simulink model "NHS_simulink_1024nfft_buffer_2017a"  (R2017a)
settings: Solver=FixedStepDiscrete  StartTime=0.0  StopTime=inf  RelTol=1e-3
libraries: simulink x2, audiosources x1, dspsnks4 x1, dspxfrm3 x1, dspvision x1
settings Model: Creator=zhouyiliang  LastModifiedBy=zhouyiliang
settings SolverCC: AutoInsertRateTranBlk=on
settings DataIOCC: LimitDataPoints=on  SaveOutput=off  SignalLogging=off  SaveTime=off  ReturnWorkspaceOutputs=on
settings OptimizationCC: LifeSpan=inf
settings DebuggingCC: AlgebraicLoopMsg=error  SingleTaskRateTransMsg=error  AllowSymbolicDim=off  SFUnexpectedBacktrackingDiag=warning  SFNoUnconditionalDefaultTransitionDiag=warning  SFExecutionAtInitializationDiag=none
settings GRTTargetCC: TargetLangStandard=C89/C90 (ANSI)
settings ConfigComp: CovMetricSettings=dw  CovSaveCumulativeToWorkspaceVar=on  CovSaveSingleToWorkspaceVar=on  CovExternalEMLEnable=off  CovSFcnEnable=off

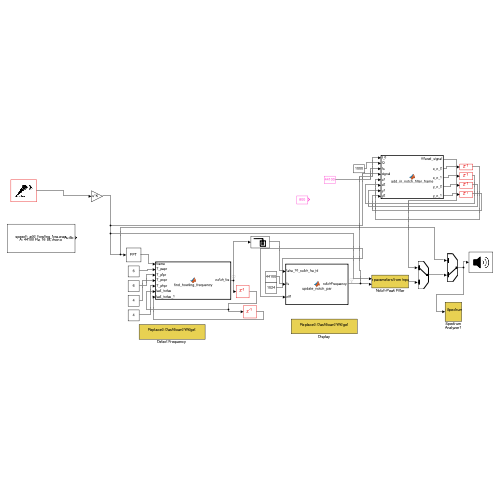
[thumbnail: Simulink's stored preview of the top-level diagram]
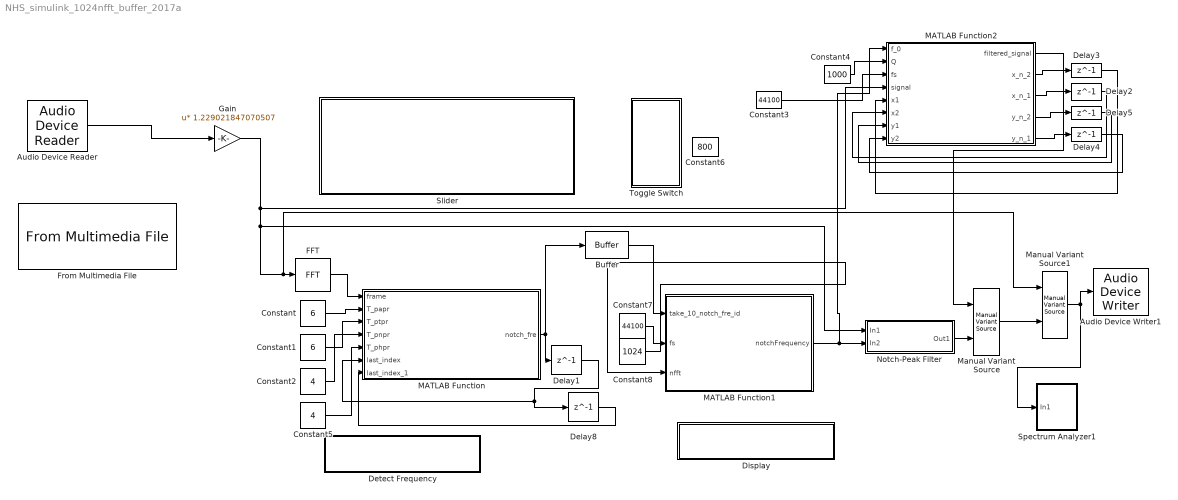
== system NHS_simulink_1024nfft_buffer_2017a ==
  Audio Device Reader : audiosources/Audio Device Reader  Driver=CoreAudio  Device=External Microphone  SampleRate=44100  NumChannels=1  SamplesPerFrame=882  BitDepth=16-bit integer  NumBuffers=10  DefaultInputChannelMapping=on  InputChannelMapping=1:2  OutputNumOverrunSamples=off  OutputDataType=double  DriverIdx=5  DeviceWarnFlag=''
  Audio Device Writer1 : dspsnks4/Audio Device Writer  Driver=CoreAudio  Device=External Headphones  InheritSampleRate=on  SampleRate=44100  BitDepth=16-bit integer  BufferSize=4096  NumBuffers=10  DefaultOutputChannelMapping=on  OutputChannelMapping=1:2  OutputNumUnderrunSamples=off  DriverIdx=5  DeviceWarnFlag=''
  Buffer : Buffer  N=5  OutputFrames=off
  Constant : Constant  Value=6
  Constant1 : Constant  Value=6
  Constant2 : Constant  Value=4
  Constant3 : Constant  Value=44100
  Constant4 : Constant  Value=1000
  Constant5 : Constant  Value=4
  Constant6 : Constant  Value=800
  Constant7 : Constant  Value=44100
  Constant8 : Constant  Value=1024
  Delay{1..5,8} (6 alike) : Delay  DelayLength=1  InitialCondition=0
  "Detect Frequency " : Subsystem  Description=Replaced Block  mask(Replaced Block){}
      mask help: This block has been replaced with an empty subsystem because it used functionality that is unavailable in Simulink R2017a.
      mask Display: fprintf('Replaced: %s\n','Dashboard Widget')
  Display : Subsystem  Description=Replaced Block  mask(Replaced Block){}
      mask help: This block has been replaced with an empty subsystem because it used functionality that is unavailable in Simulink R2017a.
      mask Display: fprintf('Replaced: %s\n','Dashboard Widget')
  FFT : dspxfrm3/FFT  FFTImplementation=Auto  CompMethod=Table lookup  TableOpt=NEW  TableOptActive=Speed  BitRevOrder=off  Normalize=off  InheritFFTLength=off  FFTLength=1024  WrapInput=on  roundingMode=Floor  overflowMode=off  firstCoeffDataTypeStr=Inherit: Same word length as input  firstCoeffLastDataTypeStr=Inherit: Same word length as input  outputMin=[]  outputMax=[]
  From Multimedia File : dspvision/From Multimedia File  inputFilename=/Users/zhouyiliang/Desktop/work/sound_output/speech_add_howling_fyra.wav  loop=on  numPlays=inf  outputStreams=Audio only  videoDataType=single  audioDataType=double  inheritSampleTime=on  userDefinedSampleTime=1/30  noAudioOutput=off  isIntensityVideo=off  fourcc=RGB  colorVideoFormat=Separate color signals  outputEOF=off  dataOrg=Column-major  audioFrameSize=882  computeAudioFrameSize=off  outSamplingMode=Sample based
  Gain : Gain  Gain=1.229021847070507  Multiplication=Matrix(u*K)
  MATLAB Function : MATLAB Function  TreatAsAtomicUnit=on
  MATLAB Function1 : MATLAB Function  TreatAsAtomicUnit=on
  MATLAB Function2 : MATLAB Function  TreatAsAtomicUnit=on
  Manual Variant Source : simulink/Signal Routing/Manual Variant Source  NumChoices=2  OverrideUsingVariant=V_1
  Manual Variant Source1 : simulink/Signal Routing/Manual Variant Source  NumChoices=2  OverrideUsingVariant=V_2
  Notch-Peak Filter : Subsystem  Description=Replaced Block  InitFcn=error('This block was designed with a newer version of Simulink. Unfortunately, your Simulink version does not support these features.')  mask(Replaced Block){}
      mask help: This block has been replaced with an empty subsystem because it used functionality that is unavailable in Simulink R2017a.
      mask Display: fprintf('Replaced: %s\n','Specifying tunable parameters from input ports supported in R2018a')
  Slider : Subsystem  DialogController=hmiCreateDDGDialog  IsWebBlock=on  mask(MWDashboardBlock){webBlockId=bec0057f-2732-4f60-8ecc-0ddb8d2f5a2f, webBlockType=slider, ShowInLibBrowser=on, ShowInitialText=on, HMISrcModelName=NHS_simulink_1024nfft_buffer_2017a}
      mask prompts: webBlockId "WebBlock Id"; webBlockType "WebBlock Type"; HMISrcModelName "Source Model"
      mask help: Set value to tune parameters or variables.
      mask Help: helpview([docroot '/mapfiles/simulink.map'], 'hmi_slider')
      mask Display:
      | if strcmp(get_param(bdroot(gcb),'BlockDiagramType'),'library')
      |  image([(matlabroot) '/toolbox/simulink/hmi/icons/Slider.png'])
      | end
  Spectrum Analyzer1 : Subsystem  Description=Replaced Block  mask(Replaced Block){}
      mask help: This block has been replaced with an empty subsystem because it used functionality that is unavailable in Simulink R2017a.
      mask Display: fprintf('Replaced: %s\n','SpectrumAnalyzer')
  Toggle Switch : Subsystem  DialogController=hmiCreateDDGDialog  IsWebBlock=on  mask(MWDashboardBlock){webBlockId=04cc992a-a373-4357-83c5-108d627a7a1e, webBlockType=toggleswitch, ShowInLibBrowser=on, ShowInitialText=on, HMISrcModelName=NHS_simulink_1024nfft_buffer_2017a}
      mask prompts: webBlockId "WebBlock Id"; webBlockType "WebBlock Type"; HMISrcModelName "Source Model"
      mask help: Set on/off value to tune parameters or variables.
      mask Help: helpview([docroot '/mapfiles/simulink.map'], 'hmi_switch')
      mask Display:
      | if strcmp(get_param(bdroot(gcb),'BlockDiagramType'),'library')
      |  image([(matlabroot) '/toolbox/simulink/hmi/icons/ToggleSwitch.png'])
      | end
  wires:
  FFT/1 -> MATLAB Function/1(frame)
  Constant/1 -> MATLAB Function/2(T_papr)
  Constant1/1 -> MATLAB Function/3(T_ptpr)
  Constant2/1 -> MATLAB Function/4(T_pnpr)
  Constant5/1 -> MATLAB Function/5(T_phpr)
  Manual Variant Source/1 -> Manual Variant Source1/2
  Delay1/1 -> Delay8/1, MATLAB Function/6(last_index)
  Notch-Peak Filter/1(Out1) -> Manual Variant Source/2
  MATLAB Function2/1(filtered_signal) -> Manual Variant Source/1
  Constant7/1 -> MATLAB Function1/2(fs)
  Constant8/1 -> MATLAB Function1/3(nfft)
  MATLAB Function1/1(notchFrequency) -> MATLAB Function2/1(f_0), Notch-Peak Filter/2(In2)
  MATLAB Function2/3(x_n_1) -> Delay2/1
  MATLAB Function2/2(x_n_2) -> Delay3/1
  MATLAB Function2/5(y_n_1) -> Delay4/1
  MATLAB Function2/4(y_n_2) -> Delay5/1
  Delay2/1 -> MATLAB Function2/6(x2)
  Delay3/1 -> MATLAB Function2/5(x1)
  Delay5/1 -> MATLAB Function2/7(y1)
  Delay4/1 -> MATLAB Function2/8(y2)
  MATLAB Function/1(notch_fre) -> Delay1/1, Buffer/1
  Delay8/1 -> MATLAB Function/7(last_index_1)
  Constant3/1 -> MATLAB Function2/3(fs)
  Constant4/1 -> MATLAB Function2/2(Q)
  Manual Variant Source1/1 -> Spectrum Analyzer1/1(In1), Audio Device Writer1/1
  Gain/1 -> Manual Variant Source1/1, FFT/1, Notch-Peak Filter/1(In1), MATLAB Function2/4(signal)
  Buffer/1 -> MATLAB Function1/1(take_10_notch_fre_id)
  Audio Device Reader/1 -> Gain/1

== system NHS_simulink_1024nfft_buffer_2017a/Detect Frequency  ==

== system NHS_simulink_1024nfft_buffer_2017a/Display ==

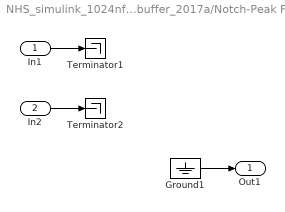
== system NHS_simulink_1024nfft_buffer_2017a/Notch-Peak Filter ==
  In1 : Inport
  In2 : Inport  Port=2
  Ground1 : Ground
  Terminator1 : Terminator
  Terminator2 : Terminator
  Out1 : Outport
  wires:
  Ground1/1 -> Out1/1
  In2/1 -> Terminator2/1
  In1/1 -> Terminator1/1

== system NHS_simulink_1024nfft_buffer_2017a/Slider ==

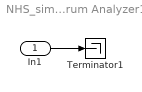
== system NHS_simulink_1024nfft_buffer_2017a/Spectrum Analyzer1 ==
  In1 : Inport
  Terminator1 : Terminator
  wires:
  In1/1 -> Terminator1/1

== system NHS_simulink_1024nfft_buffer_2017a/Toggle Switch ==

== matlab function NHS_simulink_1024nfft_buffer_2017a/MATLAB Function1 ==
  data: take_10_notch_fre_id input; notchFrequency output; fs input; nfft input
function notchFrequency = update_notch_par(take_10_notch_fre_id, fs, nfft)
    current_notch_fre_id = 2;
    if any(take_10_notch_fre_id == 2)
        notchFrequency = 0;
    else
        % 计算A中每个元素出现的次数
        [counts, bins] = histcounts(take_10_notch_fre_id);

        % 找到出现次数最大的元素的索引
        [max_count, max_idx] = max(counts);

        % 判断最大出现次数是否大于等于3，如果是，则将b赋值为对应的元素
        if max_count >= 3
            current_notch_fre_id = bins(max_idx);
        else
            current_notch_fre_id = 1;
        end
    
        freqs = linspace(0, fs, nfft);
    %     if current_notch_fre_id == 0 
    %         current_notch_fre_id = 2 ;
    %     end
        if current_notch_fre_id > 0 && current_notch_fre_id <= length(freqs)
            notchFrequency =floor(floor(max(freqs(current_notch_fre_id+1) + 20, 0)));
        else
            notchFrequency = 0;
        end
    end
end

== matlab function NHS_simulink_1024nfft_buffer_2017a/MATLAB Function ==
  data: frame input; T_papr input; T_ptpr input; T_pnpr input; T_phpr input; last_index input; notch_fre output; last_index_1 input
function notch_fre = find_howling_frequency(frame, T_papr, T_ptpr, T_pnpr,T_phpr,last_index, last_index_1)
    
%%%%%Args:
        %frame: Spectrum of one frame.
        %T_...: Power threshold value in dB for different methods.
    %Returns:
        %Notch Frequency for current frame
    power = abs(frame).^2;
    papr = zeros(length(power),1);
    avarage = mean(power);
    ret_papr = [];
    ret_ptpr = [];
    ret_pnpr = [];
    ret_phpr = [];
    for i = 4:1:length(frame)-3 % take 4:end-3
        papr(i) = 10*log10(power(i)/avarage) ;
%%%%% Peak-to-Avarage Power Ratio (PAPR)
        if papr(i) > T_papr
            ret_papr = [ret_papr, i];
        end
%%%%% Peak-to-Threshold Power Ratio (PTPR)
        if (10*log10(power(i)) > T_ptpr)
            ret_ptpr = [ret_ptpr, i];
        end
%%%%% Peak-to-Neighboring Power Ratio (PNPR)
        if (10*log10(power(i)/power(i-2)) > T_pnpr) ...
            && (10*log10(power(i)/power(i-3)) > T_pnpr)...
            && (10*log10(power(i)/power(i+2)) > T_pnpr )...
            && (10*log10(power(i)/power(i+3)) > T_pnpr)
            ret_pnpr = [ret_pnpr, i];
        end
    end
    % %%%%% Peak-to-Harmonic Power Ratio (PHPR)
    for i = 1:1:floor(length(frame)/3)
        if (10*log10(power(i)/power(2*i)) > T_phpr) && (10*log10(power(i)/power(3*i)) > T_phpr)
            ret_phpr = [ret_phpr, i];
        end
    end
    
    % interselect 
    
    fre_index = intersect(intersect(intersect(ret_papr,ret_ptpr,'stable'),ret_pnpr,'stable'),ret_phpr,'stable');
    if ~isempty(fre_index) 
        fre_index_1 = min(fre_index);
    else
%         fre_index_1 = fre_index_1+1;
        fre_index_1 = 1;
    end

    if fre_index_1 ~= last_index && fre_index_1 ~= last_index_1 
        notch_fre = fre_index_1;
    else
        notch_fre = last_index;
    end

end

== matlab function NHS_simulink_1024nfft_buffer_2017a/MATLAB Function2 ==
  data: f_0 input; Q input; fs input; filtered_signal output; x_n_2 output; signal input; x1 input; x2 input; x_n_1 output; y_n_2 output; y1 input; y2 input; y_n_1 output
function [filtered_signal,x_n_2, x_n_1, y_n_2, y_n_1] = add_iir_notch_filter_frame(f_0, Q, fs,signal, x1 ,x2, y1, y2)
    % ARG: f_0 center Frequency, Q: quality factor, fs: sampling frequency,
    % original signal
    % RETURN: filtered signal 
    if f_0 == 0
        x_n_1 = signal(end);%x(n-1)
        x_n_2 = signal(end-1); %x(n-2)
        y = [y1; y2 ;signal];
        filtered_signal=y(3:884);
        y_n_2 = y(end-1); %the one before last, y(n-2)
        y_n_1 = y(end); %last sample , y(n-1)
    else
        x_n_1 = signal(end);%x(n-1)
        x_n_2 = signal(end-1); %x(n-2)
        dw = 1; %3 dB bandwidth
        w_0 = 2*pi*f_0/fs;
        b = 1/(1+tan(dw/2)); % formula reference: help dsp.NotchPeakFilter
%         notch_b = b * [1, -2*cos(w_0) ,1]; %numerator
%         notch_a = [1, -2*b*cos(w_0), 2*b-1]; %denominator 
        N=length(signal);
        x = [x1 ;x2;signal];
        y = zeros(length(signal),1);
        y = [y1; y2 ;y];
           
        mu = 0.001;
        for k=1:N
            %%%% sng-sng LMS %%%%% to get optimized b
            %ADAPTIVE HOWLING CANCELLER USING ADAPTIVE IIR NOTCH FILTER: SIMULATION AND IMPLIMENTATION 
            %W. Leotwassana, R. Punchalard, and K Silaphan  
            notch_b = b * [1, -2*cos(w_0) ,1]; %numerator
            notch_a = [1, -2*b*cos(w_0), 2*b-1]; %denominator 
            W = [notch_b,-notch_a(2:3)]'; % notch filter coefficients
            y(k+2) = [x(k+2) x(k+1) x(k) y(k+1) y(k)] * W;%convolution with filter coefficients
            w = [1 (-0.95)]';
            g = [y(k+2) x(k+2)] * w; %g(n) is the gradient signal, g>0 the signal is increasing
            dw = dw + mu * sign(sign(abs(y(k+1))-abs(y(k)))*g); % dw decrease , filter is with less amplitue
            dw = min(dw,0.4*pi);
            dw = max(dw, 0.001);
            b = 1/(1+tan(dw/2));
            
        end
        filtered_signal=y(3:884);
        y_n_2 = y(end-1); %the one before last, y(n-2)
        y_n_1 = y(end); %last sample , y(n-1)
    
    end
end
